simulink model "Fuel_Pump_V3_1_20201113_20KHz"  (R2019b)
settings: configuration reference "Configuration" (kept outside this file)
PreLoadFcn:
  | RTWConfigurationCB('preloadfcn', bdroot);
values from neighbouring files (symbols this model uses):
  MotorPara_Base_Frq = 666.0    [fuel_pump_V3_1_20201113_20kHz.sldd]
  MotorPara_Base_I = 50.0    [fuel_pump_V3_1_20201113_20kHz.sldd]
  MotorPara_Base_RPM = 12000.0    [fuel_pump_V3_1_20201113_20kHz.sldd]
  MotorPara_Base_V = 28.0    [fuel_pump_V3_1_20201113_20kHz.sldd]
  MotorPara_Ld = 1.287E-5    [fuel_pump_V3_1_20201113_20kHz.sldd]
  MotorPara_Lq = 2.052E-5    [fuel_pump_V3_1_20201113_20kHz.sldd]
  MotorPara_Ls = 8.3475E-5    [fuel_pump_V3_1_20201113_20kHz.sldd]
  MotorPara_P = 4.0    [fuel_pump_V3_1_20201113_20kHz.sldd]
  MotorPara_Rs = 0.01638    [fuel_pump_V3_1_20201113_20kHz.sldd]
  TPBRD_HALF = 1875.0    [fuel_pump_V3_1_20201113_20kHz.sldd]
  Ts_1kHz = 0.001    [fuel_pump_V3_1_20201113_20kHz.sldd]
  Ts_200Hz = 0.005    [fuel_pump_V3_1_20201113_20kHz.sldd]
  Ts_20KHz = 5.0E-5    [fuel_pump_V3_1_20201113_20kHz.sldd]
  Ts_40Hz = 0.025    [fuel_pump_V3_1_20201113_20kHz.sldd]
  Ts_50Hz = 0.02    [fuel_pump_V3_1_20201113_20kHz.sldd]
undefined symbols (not defined in the file or in its folder): DiscIntNeverNeededParam, Down, Up
libraries: c280xlib x22, c2833xlib x6, c2837xDlib x4, c28xdmclib x4, etargetslib x4, dspstat3 x2, c2000lib x1, idelinklib_common x1
(part 3 of 4)

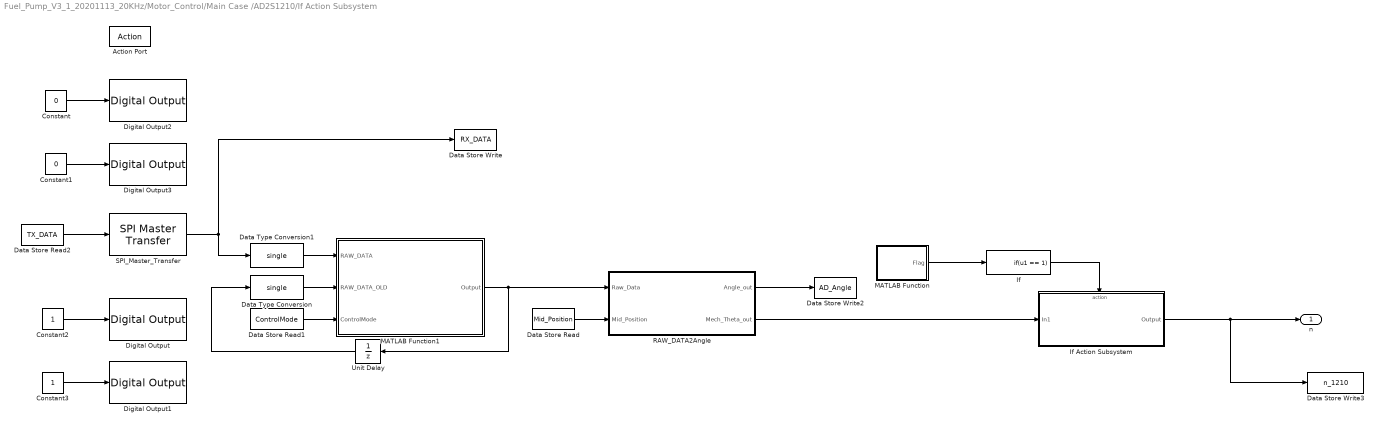
== system Fuel_Pump_V3_1_20201113_20KHz/Motor_Control/Main Case /AD2S1210/If Action Subsystem ==
  Action Port : ActionPort  ActionPortLabel=if(u1 > 0)
  Constant : Constant  Priority=1  Value=0  SampleTime=-1
  Constant1 : Constant  Priority=3  Value=0  SampleTime=-1
  Constant2 : Constant  Priority=11  SampleTime=-1
  Constant3 : Constant  Priority=12  SampleTime=-1
  Data Store Read : DataStoreRead  DataStoreName=Mid_Position
  Data Store Read1 : DataStoreRead  DataStoreName=ControlMode
  Data Store Read2 : DataStoreRead  Priority=5  DataStoreName=TX_DATA
  Data Store Write : DataStoreWrite  DataStoreName=RX_DATA
  Data Store Write2 : DataStoreWrite  DataStoreName=AD_Angle
  Data Store Write3 : DataStoreWrite  DataStoreName=n_1210
  Data Type Conversion : DataTypeConversion  OutDataTypeStr=single
  Data Type Conversion1 : DataTypeConversion  OutDataTypeStr=single
  Digital Output : c2837xDlib/Digital Output  GPIO_Number=GPIO16~GPIO23  GPIO_Bit0=off  GPIO_BIT0_Toggle=off  GPIO_Bit1=off  GPIO_BIT1_Toggle=off  GPIO_Bit2=off  GPIO_BIT2_Toggle=off  GPIO_Bit3=on  GPIO_BIT3_Toggle=off  GPIO_Bit4=off  GPIO_BIT4_Toggle=off  GPIO_Bit5=off  GPIO_BIT5_Toggle=off  GPIO_Bit6=off  GPIO_BIT6_Toggle=off  GPIO_Bit7=off  GPIO_BIT7_Toggle=off
      settings: SourceProductName=Embedded Coder Support Package for Texas Instruments C2000 Processors  SourceProductBaseCode=TIC2000
  Digital Output1 : c2837xDlib/Digital Output  GPIO_Number=GPIO16~GPIO23  GPIO_Bit0=off  GPIO_BIT0_Toggle=off  GPIO_Bit1=off  GPIO_BIT1_Toggle=off  GPIO_Bit2=off  GPIO_BIT2_Toggle=off  GPIO_Bit3=off  GPIO_BIT3_Toggle=off  GPIO_Bit4=on  GPIO_BIT4_Toggle=off  GPIO_Bit5=off  GPIO_BIT5_Toggle=off  GPIO_Bit6=off  GPIO_BIT6_Toggle=off  GPIO_Bit7=off  GPIO_BIT7_Toggle=off
      settings: SourceProductName=Embedded Coder Support Package for Texas Instruments C2000 Processors  SourceProductBaseCode=TIC2000
  Digital Output2 : c2837xDlib/Digital Output  GPIO_Number=GPIO16~GPIO23  GPIO_Bit0=off  GPIO_BIT0_Toggle=off  GPIO_Bit1=off  GPIO_BIT1_Toggle=off  GPIO_Bit2=off  GPIO_BIT2_Toggle=off  GPIO_Bit3=on  GPIO_BIT3_Toggle=off  GPIO_Bit4=off  GPIO_BIT4_Toggle=off  GPIO_Bit5=off  GPIO_BIT5_Toggle=off  GPIO_Bit6=off  GPIO_BIT6_Toggle=off  GPIO_Bit7=off  GPIO_BIT7_Toggle=off
      settings: SourceProductName=Embedded Coder Support Package for Texas Instruments C2000 Processors  SourceProductBaseCode=TIC2000
  Digital Output3 : c2837xDlib/Digital Output  GPIO_Number=GPIO16~GPIO23  GPIO_Bit0=off  GPIO_BIT0_Toggle=off  GPIO_Bit1=off  GPIO_BIT1_Toggle=off  GPIO_Bit2=off  GPIO_BIT2_Toggle=off  GPIO_Bit3=off  GPIO_BIT3_Toggle=off  GPIO_Bit4=on  GPIO_BIT4_Toggle=off  GPIO_Bit5=off  GPIO_BIT5_Toggle=off  GPIO_Bit6=off  GPIO_BIT6_Toggle=off  GPIO_Bit7=off  GPIO_BIT7_Toggle=off
      settings: SourceProductName=Embedded Coder Support Package for Texas Instruments C2000 Processors  SourceProductBaseCode=TIC2000
  If : If  IfExpression=u1 == 1  ShowElse=off
  If Action Subsystem : Subsystem  TreatAsAtomicUnit=on
  MATLAB Function : MATLAB Function  TreatAsAtomicUnit=on
  MATLAB Function1 : MATLAB Function  TreatAsAtomicUnit=on
  "RAW_DATA2Angle " : MATLAB Function  TreatAsAtomicUnit=on
  SPI_Master_Transfer : c280xlib/SPI Master Transfer  Priority=6  SPISelect=SPI_A  ClockPolarity=Rising_edge  ClockPhase=No_delay  SPIModule=uint32(0)  Mode=Master  BusSpeed=uint32(1000000)  FirstBitToTransfer=Most significant bit (MSB)  ClockMode=0  BlockFunction=Transfer  EnableRegisterAddress=off  RegisterAddress=255  OutputDataType=int8  OutputDataLength=1  DataBits=16  UseCustomSSPin=Provided by the SPI peripheral  ActiveLowSSPin=Active low  Pin=1
      settings: SourceProductName=Embedded Coder Support Package for Texas Instruments C2000 Processors  SourceProductBaseCode=TIC2000
  Unit Delay : UnitDelay  SampleTime=-1  HasFrameUpgradeWarning=on
  n : Outport
  wires:
  Constant1/1 -> Digital Output3/1
  Constant3/1 -> Digital Output1/1
  Constant/1 -> Digital Output2/1
  SPI_Master_Transfer/1 -> Data Type Conversion1/1, Data Store Write/1
  Constant2/1 -> Digital Output/1
  "RAW_DATA2Angle "/1(Angle_out) -> Data Store Write2/1
  Data Store Read2/1 -> SPI_Master_Transfer/1
  "RAW_DATA2Angle "/2(Mech_Theta_out) -> If Action Subsystem/1(In1)
  Data Store Read/1 -> "RAW_DATA2Angle "/2(Mid_Position)
  MATLAB Function/1(Flag) -> If/1
  If/1 -> If Action Subsystem/Action
  If Action Subsystem/1(Output) -> Data Store Write3/1, n/1
  MATLAB Function1/1(Output) -> "RAW_DATA2Angle "/1(Raw_Data), Unit Delay/1
  Unit Delay/1 -> Data Type Conversion/1
  Data Type Conversion/1 -> MATLAB Function1/2(RAW_DATA_OLD)
  Data Type Conversion1/1 -> MATLAB Function1/1(RAW_DATA)
  Data Store Read1/1 -> MATLAB Function1/3(ControlMode)

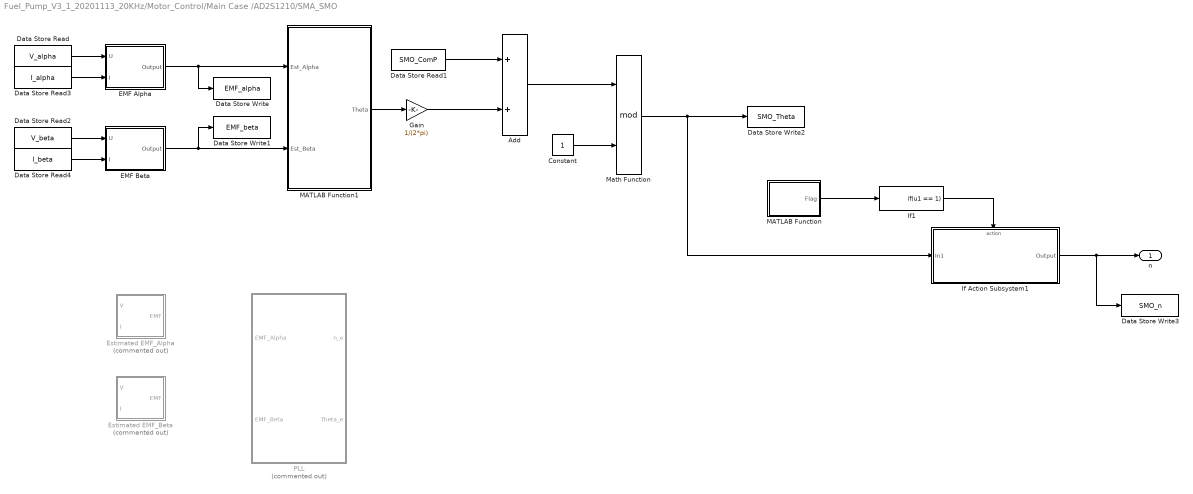
== system Fuel_Pump_V3_1_20201113_20KHz/Motor_Control/Main Case /AD2S1210/SMA_SMO ==
  Add : Sum
  Constant : Constant  OutDataTypeStr=single  SampleTime=-1
  Data Store Read : DataStoreRead  DataStoreName=V_alpha
  Data Store Read1 : DataStoreRead  DataStoreName=SMO_ComP
  Data Store Read2 : DataStoreRead  DataStoreName=V_beta
  Data Store Read3 : DataStoreRead  DataStoreName=I_alpha
  Data Store Read4 : DataStoreRead  DataStoreName=I_beta
  Data Store Write : DataStoreWrite  DataStoreName=EMF_alpha
  Data Store Write1 : DataStoreWrite  DataStoreName=EMF_beta
  Data Store Write2 : DataStoreWrite  DataStoreName=SMO_Theta
  Data Store Write3 : DataStoreWrite  DataStoreName=SMO_n
  EMF Alpha : Subsystem
  EMF Beta : Subsystem
  Estimated EMF_Alpha : Subsystem  Commented=on
  Estimated EMF_Beta : Subsystem  Commented=on
  Gain : Gain  Gain=1/(2*pi)
  If Action Subsystem1 : Subsystem  TreatAsAtomicUnit=on
  If1 : If  IfExpression=u1 == 1  ShowElse=off
  MATLAB Function : MATLAB Function  TreatAsAtomicUnit=on
  MATLAB Function1 : MATLAB Function  TreatAsAtomicUnit=on
  Math Function : Math  Operator=mod  SignedPower=off  SaturateOnIntegerOverflow=on
  PLL : Subsystem  Commented=on
  n : Outport
  wires:
  If Action Subsystem1/1(Output) -> Data Store Write3/1, n/1
  MATLAB Function/1(Flag) -> If1/1
  Data Store Read3/1 -> EMF Alpha/2(I)
  EMF Alpha/1(Output) -> MATLAB Function1/1(Est_Alpha), Data Store Write/1
  Data Store Read/1 -> EMF Alpha/1(U)
  EMF Beta/1(Output) -> MATLAB Function1/2(Est_Beta), Data Store Write1/1
  If1/1 -> If Action Subsystem1/Action
  Data Store Read4/1 -> EMF Beta/2(I)
  Data Store Read2/1 -> EMF Beta/1(U)
  Constant/1 -> Math Function/2
  Data Store Read1/1 -> Add/1
  Add/1 -> Math Function/1
  MATLAB Function1/1(Theta) -> Gain/1
  Gain/1 -> Add/2
  Math Function/1 -> If Action Subsystem1/1(In1), Data Store Write2/1

== system Fuel_Pump_V3_1_20201113_20KHz/Motor_Control/Main Case /Current_PI/PID_Id  ==
  Ref : Inport
  Fbk : Inport  Port=2
  Data Store Read : DataStoreRead  DataStoreName=PK_KpId
  Data Store Read1 : DataStoreRead  DataStoreName=uiId
  Data Store Write : DataStoreWrite  DataStoreName=uiId
  "Integral " : Subsystem
  Product : Product  OutDataTypeStr=Inherit: Same as first input
  Saturation : Saturate  UpperLimit=MotorPara_Base_V  LowerLimit=-MotorPara_Base_V
  Sum1 : Sum
  Sum2 : Sum  Inputs=+-  OutDataTypeStr=Inherit: Inherit via back propagation
  Out : Outport
  wires:
  Data Store Read1/1 -> "Integral "/1(OLD_UI)
  Fbk/1 -> Sum2/2
  Ref/1 -> Sum2/1
  Product/1 -> Sum1/1
  Data Store Read/1 -> Product/2
  "Integral "/1(UI) -> Data Store Write/1, Sum1/2
  Sum2/1 -> "Integral "/2(UP), Product/1
  Sum1/1 -> Saturation/1
  Saturation/1 -> Out/1

== system Fuel_Pump_V3_1_20201113_20KHz/Motor_Control/Main Case /Current_PI/PID_Iq ==
  Ref : Inport
  Fbk : Inport  Port=2
  Data Store Read : DataStoreRead  DataStoreName=PK_KpIq
  Data Store Read1 : DataStoreRead  DataStoreName=uiIq
  Data Store Write : DataStoreWrite  DataStoreName=uiIq
  "Integral " : Subsystem
  Product : Product  OutDataTypeStr=Inherit: Same as first input
  Saturation : Saturate  UpperLimit=MotorPara_Base_V  LowerLimit=-MotorPara_Base_V
  Sum1 : Sum
  Sum2 : Sum  Inputs=+-  OutDataTypeStr=Inherit: Inherit via back propagation
  Out : Outport
  wires:
  Data Store Read1/1 -> "Integral "/1(OLD_UI)
  Fbk/1 -> Sum2/2
  Ref/1 -> Sum2/1
  Product/1 -> Sum1/1
  Data Store Read/1 -> Product/2
  "Integral "/1(UI) -> Data Store Write/1, Sum1/2
  Sum2/1 -> "Integral "/2(UP), Product/1
  Sum1/1 -> Saturation/1
  Saturation/1 -> Out/1

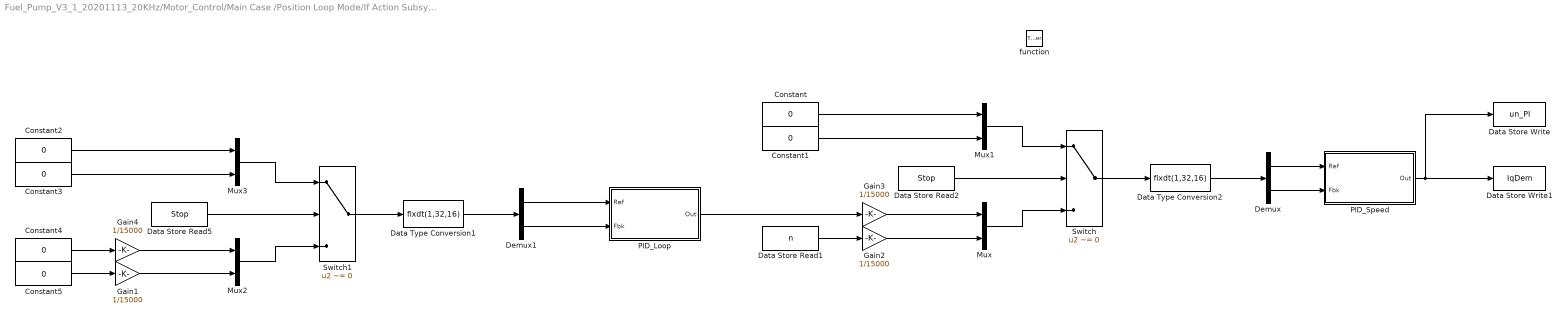
== system Fuel_Pump_V3_1_20201113_20KHz/Motor_Control/Main Case /Position Loop Mode/If Action Subsystem ==
  function : TriggerPort  TriggerType=function-call  VariantControl=Variant
  Constant{,1..5} (6 alike) : Constant  Value=0  OutDataTypeStr=single  SampleTime=-1
  Data Store Read1 : DataStoreRead  DataStoreName=n
  Data Store Read2 : DataStoreRead  DataStoreName=Stop
  Data Store Read5 : DataStoreRead  DataStoreName=Stop
  Data Store Write : DataStoreWrite  DataStoreName=un_PI
  Data Store Write1 : DataStoreWrite  DataStoreName=IqDem
  Data Type Conversion1 : DataTypeConversion  OutDataTypeStr=fixdt(1,32,16)
  Data Type Conversion2 : DataTypeConversion  OutDataTypeStr=fixdt(1,32,16)
  Demux : Demux  Outputs=2
  Demux1 : Demux  Outputs=2
  Gain{1..4} (4 alike) : Gain  Gain=1/15000  OutDataTypeStr=Inherit: Inherit via back propagation
  Mux{,1..3} (4 alike) : Mux  Inputs=2
  PID_Loop : Subsystem
  PID_Speed : Subsystem
  Switch : Switch  Criteria=u2 ~= 0
  Switch1 : Switch  Criteria=u2 ~= 0
  wires:
  PID_Speed/1(Out) -> Data Store Write1/1, Data Store Write/1
  Demux/1 -> PID_Speed/1(Ref)
  Demux/2 -> PID_Speed/2(Fbk)
  Switch/1 -> Data Type Conversion2/1
  Data Store Read2/1 -> Switch/2
  Gain3/1 -> Mux/1
  Data Store Read1/1 -> Gain2/1
  PID_Loop/1(Out) -> Gain3/1
  Gain2/1 -> Mux/2
  Mux1/1 -> Switch/1
  Mux/1 -> Switch/3
  Constant/1 -> Mux1/1
  Constant1/1 -> Mux1/2
  Data Type Conversion2/1 -> Demux/1
  Data Store Read5/1 -> Switch1/2
  Constant3/1 -> Mux3/2
  Data Type Conversion1/1 -> Demux1/1
  Mux3/1 -> Switch1/1
  Gain1/1 -> Mux2/2
  Constant2/1 -> Mux3/1
  Constant5/1 -> Gain1/1
  Gain4/1 -> Mux2/1
  Constant4/1 -> Gain4/1
  Switch1/1 -> Data Type Conversion1/1
  Demux1/1 -> PID_Loop/1(Ref)
  Mux2/1 -> Switch1/3
  Demux1/2 -> PID_Loop/2(Fbk)

== system Fuel_Pump_V3_1_20201113_20KHz/Motor_Control/Main Case /SVPWM/Inverse Park Transformation ==
  D : Inport
  Q : Inport  Port=2
  theta : Inport  Port=3
  Gain : Gain  Gain=2*pi
  Product{,1..3} (4 alike) : Product  OutDataTypeStr=Inherit: Same as first input
  Sin : Trigonometry  OutputSignalType=real
  Sin1 : Trigonometry  Operator=cos  OutputSignalType=real
  Sum1 : Sum  Inputs=|++  OutDataTypeStr=Inherit: Same as first input
  Sum2 : Sum  Inputs=|+-  OutDataTypeStr=Inherit: Same as first input
  Alpha : Outport
  Beta : Outport  Port=2
  wires:
  Sin1/1 -> Product2/2, Product/2
  Sin/1 -> Product3/2, Product1/2
  Product3/1 -> Sum1/2
  Sum1/1 -> Beta/1
  D/1 -> Product3/1, Product/1
  Product2/1 -> Sum1/1
  Sum2/1 -> Alpha/1
  Product/1 -> Sum2/1
  Product1/1 -> Sum2/2
  theta/1 -> Gain/1
  Q/1 -> Product2/1, Product1/1
  Gain/1 -> Sin/1, Sin1/1

== system Fuel_Pump_V3_1_20201113_20KHz/Motor_Control/Main Case /Speed Loop Mode/If Action Subsystem ==
  function : TriggerPort  TriggerType=function-call  VariantControl=Variant
  Constant : Constant  Value=0  OutDataTypeStr=single  SampleTime=-1
  Constant1 : Constant  Value=0  OutDataTypeStr=single  SampleTime=-1
  Data Store Read1 : DataStoreRead  DataStoreName=n
  Data Store Read2 : DataStoreRead  DataStoreName=Stop
  Data Store Read3 : DataStoreRead  DataStoreName=nDem_PI
  Data Store Write1 : DataStoreWrite  DataStoreName=IqDem
  Demux : Demux  Outputs=2
  Mux : Mux  Inputs=2
  Mux1 : Mux  Inputs=2
  "PID_n " : Subsystem
  Switch : Switch  Criteria=u2 ~= 0
  wires:
  "PID_n "/1(Out) -> Data Store Write1/1
  Demux/1 -> "PID_n "/1(Ref)
  Demux/2 -> "PID_n "/2(Fbk)
  Data Store Read2/1 -> Switch/2
  Data Store Read3/1 -> Mux/1
  Data Store Read1/1 -> Mux/2
  Mux1/1 -> Switch/1
  Mux/1 -> Switch/3
  Constant/1 -> Mux1/1
  Constant1/1 -> Mux1/2
  Switch/1 -> Demux/1

== system Fuel_Pump_V3_1_20201113_20KHz/Motor_Control/Main Case /AD2S1210/If Action Subsystem/If Action Subsystem ==
  In1 : Inport
  Action Port : ActionPort  ActionPortLabel=if(u1 == 1)
  Delay1 : Delay  DelayLength=1
  First Order Filter : Subsystem
  MATLAB Function1 : MATLAB Function  TreatAsAtomicUnit=on
  Output : Outport
  wires:
  In1/1 -> Delay1/1, MATLAB Function1/1(theta)
  Delay1/1 -> MATLAB Function1/2(theta_old)
  First Order Filter/1("output ") -> Output/1
  MATLAB Function1/1(speed) -> First Order Filter/1(input)

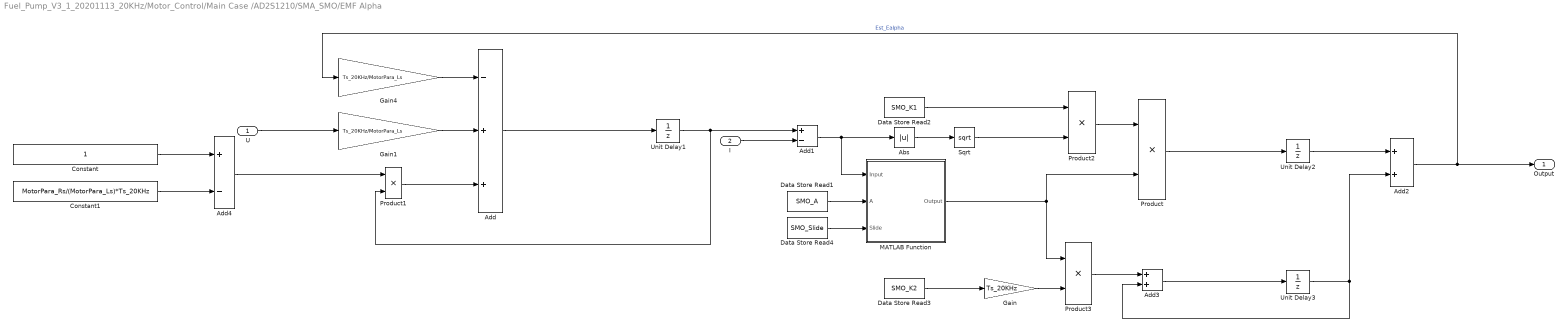
== system Fuel_Pump_V3_1_20201113_20KHz/Motor_Control/Main Case /AD2S1210/SMA_SMO/EMF Alpha ==
  U : Inport
  I : Inport  Port=2
  Abs : Abs
  Add : Sum  Inputs=-++
  Add1 : Sum  Inputs=+-  OutDataTypeStr=Inherit: Inherit via back propagation
  Add2 : Sum
  Add3 : Sum
  Add4 : Sum  Inputs=+-
  Constant : Constant  OutDataTypeStr=single  SampleTime=-1
  Constant1 : Constant  Value=MotorPara_Rs/(MotorPara_Ls)*Ts_20KHz  OutDataTypeStr=single  SampleTime=-1
  Data Store Read1 : DataStoreRead  DataStoreName=SMO_A
  Data Store Read2 : DataStoreRead  DataStoreName=SMO_K1
  Data Store Read3 : DataStoreRead  DataStoreName=SMO_K2
  Data Store Read4 : DataStoreRead  DataStoreName=SMO_Slide
  Gain : Gain  Gain=Ts_20KHz
  Gain1 : Gain  Gain=Ts_20KHz/MotorPara_Ls  OutDataTypeStr=Inherit: Inherit via back propagation
  Gain4 : Gain  Gain=Ts_20KHz/MotorPara_Ls  OutDataTypeStr=Inherit: Inherit via back propagation
  MATLAB Function : MATLAB Function  TreatAsAtomicUnit=on
  Product{,1..3} (4 alike) : Product
  Sqrt : Sqrt  SaturateOnIntegerOverflow=on
  Unit Delay1 : UnitDelay  SampleTime=-1  HasFrameUpgradeWarning=on
  Unit Delay2 : UnitDelay  SampleTime=-1  HasFrameUpgradeWarning=on
  Unit Delay3 : UnitDelay  SampleTime=-1  HasFrameUpgradeWarning=on
  Output : Outport
  wires:
  Product3/1 -> Add3/1
  Gain4/1 -> Add/1
  Gain1/1 -> Add/2
  Add2/1 -> Output/1, Gain4/1  "Est_Ealpha"
  Product1/1 -> Add/3
  Product2/1 -> Product/1
  Sqrt/1 -> Product2/2
  U/1 -> Gain1/1
  I/1 -> Add1/2
  Add1/1 -> MATLAB Function/1(Input), Abs/1
  Abs/1 -> Sqrt/1
  Unit Delay2/1 -> Add2/1
  Add4/1 -> Product1/1
  Constant/1 -> Add4/1
  Constant1/1 -> Add4/2
  Data Store Read1/1 -> MATLAB Function/2(A)
  Data Store Read2/1 -> Product2/1
  Gain/1 -> Product3/2
  Data Store Read3/1 -> Gain/1
  Unit Delay1/1 -> Product1/2, Add1/1
  Unit Delay3/1 -> Add3/2, Add2/2
  Add/1 -> Unit Delay1/1
  MATLAB Function/1(Output) -> Product/2, Product3/1
  Product/1 -> Unit Delay2/1
  Add3/1 -> Unit Delay3/1
  Data Store Read4/1 -> MATLAB Function/3(Slide)

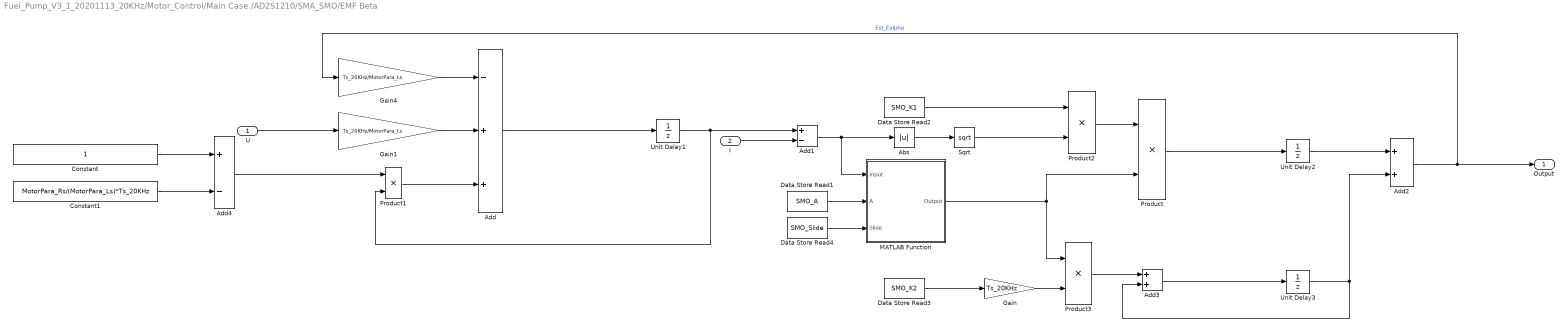
== system Fuel_Pump_V3_1_20201113_20KHz/Motor_Control/Main Case /AD2S1210/SMA_SMO/EMF Beta ==
  U : Inport
  I : Inport  Port=2
  Abs : Abs
  Add : Sum  Inputs=-++
  Add1 : Sum  Inputs=+-  OutDataTypeStr=Inherit: Inherit via back propagation
  Add2 : Sum
  Add3 : Sum
  Add4 : Sum  Inputs=+-
  Constant : Constant  OutDataTypeStr=single  SampleTime=-1
  Constant1 : Constant  Value=MotorPara_Rs/(MotorPara_Ls)*Ts_20KHz  OutDataTypeStr=single  SampleTime=-1
  Data Store Read1 : DataStoreRead  DataStoreName=SMO_A
  Data Store Read2 : DataStoreRead  DataStoreName=SMO_K1
  Data Store Read3 : DataStoreRead  DataStoreName=SMO_K2
  Data Store Read4 : DataStoreRead  DataStoreName=SMO_Slide
  Gain : Gain  Gain=Ts_20KHz
  Gain1 : Gain  Gain=Ts_20KHz/MotorPara_Ls  OutDataTypeStr=Inherit: Inherit via back propagation
  Gain4 : Gain  Gain=Ts_20KHz/MotorPara_Ls  OutDataTypeStr=Inherit: Inherit via back propagation
  MATLAB Function : MATLAB Function  TreatAsAtomicUnit=on
  Product{,1..3} (4 alike) : Product
  Sqrt : Sqrt  SaturateOnIntegerOverflow=on
  Unit Delay1 : UnitDelay  SampleTime=-1  HasFrameUpgradeWarning=on
  Unit Delay2 : UnitDelay  SampleTime=-1  HasFrameUpgradeWarning=on
  Unit Delay3 : UnitDelay  SampleTime=-1  HasFrameUpgradeWarning=on
  Output : Outport
  wires:
  Data Store Read4/1 -> MATLAB Function/3(Slide)
  Add3/1 -> Unit Delay3/1
  Product/1 -> Unit Delay2/1
  MATLAB Function/1(Output) -> Product3/1, Product/2
  Add/1 -> Unit Delay1/1
  Unit Delay3/1 -> Add2/2, Add3/2
  Unit Delay1/1 -> Add1/1, Product1/2
  Data Store Read3/1 -> Gain/1
  Gain/1 -> Product3/2
  Data Store Read2/1 -> Product2/1
  Data Store Read1/1 -> MATLAB Function/2(A)
  Constant1/1 -> Add4/2
  Constant/1 -> Add4/1
  Add4/1 -> Product1/1
  Unit Delay2/1 -> Add2/1
  Abs/1 -> Sqrt/1
  Add1/1 -> Abs/1, MATLAB Function/1(Input)
  I/1 -> Add1/2
  U/1 -> Gain1/1
  Sqrt/1 -> Product2/2
  Product2/1 -> Product/1
  Product1/1 -> Add/3
  Add2/1 -> Gain4/1, Output/1  "Est_Ealpha"
  Gain1/1 -> Add/2
  Gain4/1 -> Add/1
  Product3/1 -> Add3/1

== system Fuel_Pump_V3_1_20201113_20KHz/Motor_Control/Main Case /AD2S1210/SMA_SMO/Estimated EMF_Alpha ==
  V : Inport
  I : Inport  Port=2
  Add : Sum  Inputs=+--
  Add1 : Sum
  Add2 : Sum  Inputs=+-
  Data Store Read1 : DataStoreRead  DataStoreName=SMO_Slide
  Data Store Read2 : DataStoreRead  DataStoreName=SMO_A
  First Order Filter : Subsystem
  Gain2 : Gain  Gain=exp(-MotorPara_Rs*Ts_20KHz/MotorPara_Ls)
  Gain3 : Gain  Gain=(1/MotorPara_Rs)*(1-exp(-MotorPara_Rs*Ts_20KHz/MotorPara_Ls))
  MATLAB Function : MATLAB Function  TreatAsAtomicUnit=on
  Unit Delay : UnitDelay  SampleTime=-1  HasFrameUpgradeWarning=on
  Unit Delay1 : UnitDelay  SampleTime=-1  HasFrameUpgradeWarning=on
  Unit Delay2 : UnitDelay  SampleTime=-1  HasFrameUpgradeWarning=on
  EMF : Outport
  wires:
  First Order Filter/1("output ") -> EMF/1, Unit Delay2/1
  Gain2/1 -> Add1/2
  Add1/1 -> Unit Delay/1, Add2/1  "Est_Ialpha"
  Gain3/1 -> Add1/1
  MATLAB Function/1(output) -> Unit Delay1/1, First Order Filter/1(input)
  Data Store Read1/1 -> MATLAB Function/2(slide)
  Add/1 -> Gain3/1
  Add2/1 -> MATLAB Function/1(input)
  Unit Delay/1 -> Gain2/1  "Est_Ialpha_old"
  I/1 -> Add2/2
  Unit Delay1/1 -> Add/3  "Zalpha_old"
  Unit Delay2/1 -> Add/2  "Ealpha_old"
  V/1 -> Add/1
  Data Store Read2/1 -> MATLAB Function/3(E0)

== system Fuel_Pump_V3_1_20201113_20KHz/Motor_Control/Main Case /AD2S1210/SMA_SMO/Estimated EMF_Beta ==
  V : Inport
  I : Inport  Port=2
  Add : Sum  Inputs=+--
  Add1 : Sum
  Add2 : Sum  Inputs=+-
  Data Store Read1 : DataStoreRead  DataStoreName=SMO_Slide
  Data Store Read2 : DataStoreRead  DataStoreName=SMO_A
  First Order Filter : Subsystem
  Gain2 : Gain  Gain=exp(-MotorPara_Rs*Ts_20KHz/MotorPara_Ls)
  Gain3 : Gain  Gain=(1/MotorPara_Rs)*(1-exp(-MotorPara_Rs*Ts_20KHz/MotorPara_Ls))
  MATLAB Function : MATLAB Function  TreatAsAtomicUnit=on
  Unit Delay : UnitDelay  SampleTime=-1  HasFrameUpgradeWarning=on
  Unit Delay1 : UnitDelay  SampleTime=-1  HasFrameUpgradeWarning=on
  Unit Delay2 : UnitDelay  SampleTime=-1  HasFrameUpgradeWarning=on
  EMF : Outport
  wires:
  Data Store Read2/1 -> MATLAB Function/3(E0)
  V/1 -> Add/1
  Unit Delay2/1 -> Add/2  "Ealpha_old"
  Unit Delay1/1 -> Add/3  "Zalpha_old"
  I/1 -> Add2/2
  Unit Delay/1 -> Gain2/1  "Est_Ialpha_old"
  Add2/1 -> MATLAB Function/1(input)
  Add/1 -> Gain3/1
  Data Store Read1/1 -> MATLAB Function/2(slide)
  MATLAB Function/1(output) -> First Order Filter/1(input), Unit Delay1/1
  Gain3/1 -> Add1/1
  Add1/1 -> Add2/1, Unit Delay/1  "Est_Ialpha"
  Gain2/1 -> Add1/2
  First Order Filter/1("output ") -> Unit Delay2/1, EMF/1

== system Fuel_Pump_V3_1_20201113_20KHz/Motor_Control/Main Case /AD2S1210/SMA_SMO/If Action Subsystem1 ==
  In1 : Inport
  Action Port : ActionPort  ActionPortLabel=if(u1 == 1)
  Data Store Read : DataStoreRead  DataStoreName=n_R
  Data Store Read1 : DataStoreRead  DataStoreName=n_Q
  Delay1 : Delay  DelayLength=1
  First Order Filter : Subsystem  Commented=on
  Kalman_Filter : MATLAB Function  TreatAsAtomicUnit=on
  MATLAB Function1 : MATLAB Function  TreatAsAtomicUnit=on
  Output : Outport
  wires:
  In1/1 -> Delay1/1, MATLAB Function1/1(theta)
  MATLAB Function1/1(speed) -> Kalman_Filter/1(Input)
  Delay1/1 -> MATLAB Function1/2(theta_old)
  Kalman_Filter/1(optimal_value_out) -> Output/1
  Data Store Read1/1 -> Kalman_Filter/2(n_Q)
  Data Store Read/1 -> Kalman_Filter/3(n_R)

== system Fuel_Pump_V3_1_20201113_20KHz/Motor_Control/Main Case /AD2S1210/SMA_SMO/PLL ==
  EMF_Alpha : Inport
  EMF_Beta : Inport  Port=2
  Add : Sum  Inputs=+-
  Add1 : Sum
  Constant : Constant  Value=2*pi  OutDataTypeStr=single  SampleTime=-1
  Constant1 : Constant  OutDataTypeStr=single  SampleTime=-1
  Data Store Read : DataStoreRead  DataStoreName=SMO_ComP
  Discrete-Time Integrator : DiscreteIntegrator  SampleTime=-1  OutDataTypeStr=single  ICPrevOutput=DiscIntNeverNeededParam  ICPrevScaledInput=DiscIntNeverNeededParam
  Gain : Gain  Gain=-1
  Gain1 : Gain  Gain=1/(2*pi)
  Math Function : Math  Operator=mod  SignedPower=off  OutputSignalType=real  SaturateOnIntegerOverflow=on
  Math Function1 : Math  Operator=mod  SignedPower=off  OutputSignalType=real  SaturateOnIntegerOverflow=on
  "PLL_PI " : Subsystem
  Product : Product
  Product1 : Product
  Sin : Trigonometry  OutputSignalType=real
  Sin1 : Trigonometry  Operator=cos  OutputSignalType=real
  n_e : Outport
  Theta_e : Outport  Port=2
  wires:
  EMF_Alpha/1 -> Gain/1
  Gain/1 -> Product/2
  EMF_Beta/1 -> Product1/1
  Product/1 -> Add/1
  Product1/1 -> Add/2
  Discrete-Time Integrator/1 -> Math Function/1
  Math Function/1 -> Sin/1, Gain1/1, Sin1/1
  Constant/1 -> Math Function/2
  Sin1/1 -> Product/1
  Sin/1 -> Product1/2
  Add/1 -> "PLL_PI "/1(Ref)
  "PLL_PI "/1(Out) -> n_e/1, Discrete-Time Integrator/1
  Gain1/1 -> Add1/1
  Data Store Read/1 -> Add1/2
  Constant1/1 -> Math Function1/2
  Add1/1 -> Math Function1/1
  Math Function1/1 -> Theta_e/1

== system Fuel_Pump_V3_1_20201113_20KHz/Motor_Control/Main Case /Current_PI/PID_Id /Integral  ==
  OLD_UI : Inport
  UP : Inport  Port=2
  Data Store Read2 : DataStoreRead  DataStoreName=PK_KiId
  Gain : Gain  Gain=Ts_20KHz
  Product1 : Product  OutDataTypeStr=Inherit: Same as first input
  Sum3 : Sum
  UI : Outport
  wires:
  Sum3/1 -> UI/1
  UP/1 -> Product1/2
  Product1/1 -> Sum3/2
  OLD_UI/1 -> Sum3/1
  Data Store Read2/1 -> Gain/1
  Gain/1 -> Product1/1

== system Fuel_Pump_V3_1_20201113_20KHz/Motor_Control/Main Case /Current_PI/PID_Iq/Integral  ==
  OLD_UI : Inport
  UP : Inport  Port=2
  Data Store Read2 : DataStoreRead  DataStoreName=PK_KiIq
  Gain : Gain  Gain=Ts_20KHz
  Product1 : Product  OutDataTypeStr=Inherit: Same as first input
  Sum3 : Sum
  UI : Outport
  wires:
  Sum3/1 -> UI/1
  UP/1 -> Product1/2
  Product1/1 -> Sum3/2
  OLD_UI/1 -> Sum3/1
  Data Store Read2/1 -> Gain/1
  Gain/1 -> Product1/1

== system Fuel_Pump_V3_1_20201113_20KHz/Motor_Control/Main Case /Position Loop Mode/If Action Subsystem/PID_Loop ==
  Ref : Inport
  Fbk : Inport  Port=2
  " " : etargetslib/ 
      settings: SourceProductName=MATLAB Coder  SourceProductBaseCode=ME
  " 1" : etargetslib/ 
      settings: SourceProductName=MATLAB Coder  SourceProductBaseCode=ME
  Data Store Read : DataStoreRead  DataStoreName=PK_Kpn
  Data Store Read1 : DataStoreRead  DataStoreName=uin
  Data Store Write : DataStoreWrite  DataStoreName=en
  Data Store Write1 : DataStoreWrite  DataStoreName=uin
  Data Type Conversion{,1..2,5} (4 alike) : DataTypeConversion
  Product : Product  OutDataTypeStr=Inherit: Same as first input
  Saturation : Saturate  UpperLimit=1  LowerLimit=-1  OutDataTypeStr=Inherit: Inherit via back propagation
  Saturation1 : Saturate  UpperLimit=1  LowerLimit=-1  OutDataTypeStr=fixdt(1,32,16)
  Sum1 : Sum
  Sum2 : Sum  Inputs=+-  OutDataTypeStr=fixdt(1,32,16)
  UI_REG3 : Subsystem  AncestorBlock=c28xdmclib/PID Controller/UI_REG3
  Out : Outport
  wires:
  Data Type Conversion2/1 -> UI_REG3/1(OLD_UI_REG3)
  Data Type Conversion1/1 -> Data Store Write1/1
  UI_REG3/1(UI_REG1) -> Saturation1/1
  Sum1/1 -> Saturation/1
  Data Type Conversion5/1 -> Data Store Write/1
  Saturation/1 -> Out/1
  Saturation1/1 -> Sum1/2, Data Type Conversion1/1
  Data Type Conversion/1 -> Product/2
  Fbk/1 -> " 1"/1
  Data Store Read1/1 -> Data Type Conversion2/1
  Ref/1 -> " "/1
  Sum2/1 -> Product/1, Data Type Conversion5/1
  " 1"/1 -> Sum2/2
  " "/1 -> Sum2/1
  Product/1 -> UI_REG3/2(up_reg3), Sum1/1
  Data Store Read/1 -> Data Type Conversion/1

== system Fuel_Pump_V3_1_20201113_20KHz/Motor_Control/Main Case /Position Loop Mode/If Action Subsystem/PID_Speed ==
  Ref : Inport
  Fbk : Inport  Port=2
  " " : etargetslib/ 
      settings: SourceProductName=MATLAB Coder  SourceProductBaseCode=ME
  " 1" : etargetslib/ 
      settings: SourceProductName=MATLAB Coder  SourceProductBaseCode=ME
  Data Store Read : DataStoreRead  DataStoreName=PK_Kpn
  Data Store Read1 : DataStoreRead  DataStoreName=uin
  Data Store Write : DataStoreWrite  DataStoreName=en
  Data Store Write1 : DataStoreWrite  DataStoreName=uin
  Data Type Conversion{,1..2,5} (4 alike) : DataTypeConversion
  Product : Product  OutDataTypeStr=Inherit: Same as first input
  Saturation : Saturate  UpperLimit=1  LowerLimit=-1  OutDataTypeStr=Inherit: Inherit via back propagation
  Saturation1 : Saturate  UpperLimit=1  LowerLimit=-1  OutDataTypeStr=fixdt(1,32,16)
  Sum1 : Sum
  Sum2 : Sum  Inputs=+-  OutDataTypeStr=fixdt(1,32,16)
  UI_REG3 : Subsystem  AncestorBlock=c28xdmclib/PID Controller/UI_REG3
  Out : Outport
  wires:
  Data Store Read/1 -> Data Type Conversion/1
  Product/1 -> Sum1/1, UI_REG3/2(up_reg3)
  " "/1 -> Sum2/1
  " 1"/1 -> Sum2/2
  Sum2/1 -> Data Type Conversion5/1, Product/1
  Ref/1 -> " "/1
  Data Store Read1/1 -> Data Type Conversion2/1
  Fbk/1 -> " 1"/1
  Data Type Conversion/1 -> Product/2
  Saturation1/1 -> Data Type Conversion1/1, Sum1/2
  Saturation/1 -> Out/1
  Data Type Conversion5/1 -> Data Store Write/1
  Sum1/1 -> Saturation/1
  UI_REG3/1(UI_REG1) -> Saturation1/1
  Data Type Conversion1/1 -> Data Store Write1/1
  Data Type Conversion2/1 -> UI_REG3/1(OLD_UI_REG3)

== system Fuel_Pump_V3_1_20201113_20KHz/Motor_Control/Main Case /Speed Loop Mode/If Action Subsystem/PID_n  ==
  Ref : Inport
  Fbk : Inport  Port=2
  Data Store Read : DataStoreRead  DataStoreName=PK_Kpn
  Data Store Read1 : DataStoreRead  DataStoreName=uin
  Data Store Write : DataStoreWrite  DataStoreName=uin
  "Integral " : Subsystem
  Product : Product  OutDataTypeStr=Inherit: Same as first input
  Saturation : Saturate  UpperLimit=MotorPara_Base_I*1.5  LowerLimit=-MotorPara_Base_I*1.5
  Sum1 : Sum
  Sum2 : Sum  Inputs=+-  OutDataTypeStr=Inherit: Inherit via back propagation
  Out : Outport
  wires:
  Data Store Read1/1 -> "Integral "/1(OLD_UI)
  Fbk/1 -> Sum2/2
  Ref/1 -> Sum2/1
  Product/1 -> Sum1/1
  Data Store Read/1 -> Product/2
  "Integral "/1(UI) -> Data Store Write/1, Sum1/2
  Sum2/1 -> "Integral "/2(UP), Product/1
  Sum1/1 -> Saturation/1
  Saturation/1 -> Out/1

== system Fuel_Pump_V3_1_20201113_20KHz/Motor_Control/Main Case /AD2S1210/If Action Subsystem/If Action Subsystem/First Order Filter ==
  input : Inport
  Add : Sum  Inputs=+-
  Add3 : Sum  AccumDataTypeStr=single
  Constant : Constant  OutDataTypeStr=single  SampleTime=-1
  Data Store Read1 : DataStoreRead  DataStoreName=n_Filter
  Data Store Read2 : DataStoreRead  DataStoreName=n_Filter
  Gain : Gain  Gain=2*pi*Ts_20KHz*20
  Gain1 : Gain  Gain=2*pi*Ts_20KHz*20
  Product : Product
  Product1 : Product
  Unit Delay3 : UnitDelay  SampleTime=-1  HasFrameUpgradeWarning=on
  "output " : Outport
  wires:
  input/1 -> Product/1
  Product/1 -> Add3/1
  Product1/1 -> Unit Delay3/1
  Add3/1 -> Product1/1, "output "/1
  Unit Delay3/1 -> Add3/2
  Data Store Read2/1 -> Gain/1
  Gain/1 -> Product/2
  Data Store Read1/1 -> Gain1/1
  Add/1 -> Product1/2
  Gain1/1 -> Add/2
  Constant/1 -> Add/1

== system Fuel_Pump_V3_1_20201113_20KHz/Motor_Control/Main Case /AD2S1210/SMA_SMO/Estimated EMF_Alpha/First Order Filter ==
  input : Inport
  Add : Sum  Inputs=+-
  Add3 : Sum  AccumDataTypeStr=single
  Constant : Constant  OutDataTypeStr=single
  Data Store Read1 : DataStoreRead  DataStoreName=SMO_Filter
  Data Store Read2 : DataStoreRead  DataStoreName=SMO_Filter
  Gain : Gain  Gain=MotorPara_P/60*2*pi*Ts_20KHz
  Gain1 : Gain  Gain=MotorPara_P/60*2*pi*Ts_20KHz
  Product : Product
  Product1 : Product
  Unit Delay3 : UnitDelay  SampleTime=-1  HasFrameUpgradeWarning=on
  "output " : Outport
  wires:
  input/1 -> Product/1
  Product/1 -> Add3/1
  Product1/1 -> Unit Delay3/1
  Add3/1 -> Product1/1, "output "/1
  Unit Delay3/1 -> Add3/2
  Data Store Read2/1 -> Gain/1
  Gain/1 -> Product/2
  Data Store Read1/1 -> Gain1/1
  Add/1 -> Product1/2
  Gain1/1 -> Add/2
  Constant/1 -> Add/1

== system Fuel_Pump_V3_1_20201113_20KHz/Motor_Control/Main Case /AD2S1210/SMA_SMO/Estimated EMF_Beta/First Order Filter ==
  input : Inport
  Add : Sum  Inputs=+-
  Add3 : Sum  AccumDataTypeStr=single
  Constant : Constant  OutDataTypeStr=single
  Data Store Read1 : DataStoreRead  DataStoreName=SMO_Filter
  Data Store Read2 : DataStoreRead  DataStoreName=SMO_Filter
  Gain : Gain  Gain=MotorPara_P/60*2*pi*Ts_20KHz
  Gain1 : Gain  Gain=MotorPara_P/60*2*pi*Ts_20KHz
  Product : Product
  Product1 : Product
  Unit Delay3 : UnitDelay  SampleTime=-1  HasFrameUpgradeWarning=on
  "output " : Outport
  wires:
  Constant/1 -> Add/1
  Gain1/1 -> Add/2
  Add/1 -> Product1/2
  Data Store Read1/1 -> Gain1/1
  Gain/1 -> Product/2
  Data Store Read2/1 -> Gain/1
  Unit Delay3/1 -> Add3/2
  Add3/1 -> "output "/1, Product1/1
  Product1/1 -> Unit Delay3/1
  Product/1 -> Add3/1
  input/1 -> Product/1

== system Fuel_Pump_V3_1_20201113_20KHz/Motor_Control/Main Case /AD2S1210/SMA_SMO/If Action Subsystem1/First Order Filter ==
  input : Inport
  Add : Sum  Inputs=+-
  Add3 : Sum  AccumDataTypeStr=single
  Constant : Constant  OutDataTypeStr=single  SampleTime=-1
  Data Store Read1 : DataStoreRead  DataStoreName=n_Filter
  Data Store Read2 : DataStoreRead  DataStoreName=SMO_Filter
  Gain : Gain  Gain=2*pi*Ts_20KHz*20
  Gain1 : Gain  Gain=2*pi*Ts_20KHz*20
  Product : Product
  Product1 : Product
  Unit Delay3 : UnitDelay  SampleTime=-1  HasFrameUpgradeWarning=on
  "output " : Outport
  wires:
  input/1 -> Product/1
  Product/1 -> Add3/1
  Product1/1 -> Unit Delay3/1
  Add3/1 -> Product1/1, "output "/1
  Unit Delay3/1 -> Add3/2
  Data Store Read2/1 -> Gain/1
  Gain/1 -> Product/2
  Data Store Read1/1 -> Gain1/1
  Add/1 -> Product1/2
  Gain1/1 -> Add/2
  Constant/1 -> Add/1

== system Fuel_Pump_V3_1_20201113_20KHz/Motor_Control/Main Case /AD2S1210/SMA_SMO/PLL/PLL_PI  ==
  Ref : Inport
  Data Store Read : DataStoreRead  DataStoreName=SMO_KP
  Data Store Read1 : DataStoreRead  DataStoreName=SMO_uin
  Data Store Write1 : DataStoreWrite  DataStoreName=SMO_uin
  "Integral " : Subsystem
  Product : Product  OutDataTypeStr=Inherit: Same as first input
  Sum1 : Sum
  Out : Outport
  wires:
  Data Store Read1/1 -> "Integral "/1(OLD_UI)
  Product/1 -> Sum1/1
  Data Store Read/1 -> Product/2
  Ref/1 -> "Integral "/2(UP), Product/1
  "Integral "/1(UI) -> Data Store Write1/1, Sum1/2
  Sum1/1 -> Out/1

== system Fuel_Pump_V3_1_20201113_20KHz/Motor_Control/Main Case /Position Loop Mode/If Action Subsystem/PID_Loop/UI_REG3 ==
  OLD_UI_REG3 : Inport
  up_reg3 : Inport  Port=2
  Data Store Read : DataStoreRead  DataStoreName=PK_Kin
  Data Type Conversion : DataTypeConversion
  Product : Product  OutDataTypeStr=Inherit: Same as first input
  Sum1 : Sum  OutDataTypeStr=fixdt(1,32,16)
  UI_REG1 : Outport
  wires:
  Data Type Conversion/1 -> Product/1
  Data Store Read/1 -> Data Type Conversion/1
  up_reg3/1 -> Product/2
  Sum1/1 -> UI_REG1/1
  Product/1 -> Sum1/2
  OLD_UI_REG3/1 -> Sum1/1

== system Fuel_Pump_V3_1_20201113_20KHz/Motor_Control/Main Case /Position Loop Mode/If Action Subsystem/PID_Speed/UI_REG3 ==
  OLD_UI_REG3 : Inport
  up_reg3 : Inport  Port=2
  Data Store Read : DataStoreRead  DataStoreName=PK_Kin
  Data Type Conversion : DataTypeConversion
  Product : Product  OutDataTypeStr=Inherit: Same as first input
  Sum1 : Sum  OutDataTypeStr=fixdt(1,32,16)
  UI_REG1 : Outport
  wires:
  OLD_UI_REG3/1 -> Sum1/1
  Product/1 -> Sum1/2
  Sum1/1 -> UI_REG1/1
  up_reg3/1 -> Product/2
  Data Store Read/1 -> Data Type Conversion/1
  Data Type Conversion/1 -> Product/1

== system Fuel_Pump_V3_1_20201113_20KHz/Motor_Control/Main Case /Speed Loop Mode/If Action Subsystem/PID_n /Integral  ==
  OLD_UI : Inport
  UP : Inport  Port=2
  Data Store Read2 : DataStoreRead  DataStoreName=PK_Kin
  Gain : Gain  Gain=Ts_1kHz
  Product1 : Product  OutDataTypeStr=Inherit: Same as first input
  Sum3 : Sum
  UI : Outport
  wires:
  Sum3/1 -> UI/1
  UP/1 -> Product1/2
  Product1/1 -> Sum3/2
  OLD_UI/1 -> Sum3/1
  Data Store Read2/1 -> Gain/1
  Gain/1 -> Product1/1

== system Fuel_Pump_V3_1_20201113_20KHz/Motor_Control/Main Case /AD2S1210/SMA_SMO/PLL/PLL_PI /Integral  ==
  OLD_UI : Inport
  UP : Inport  Port=2
  Data Store Read2 : DataStoreRead  DataStoreName=SMO_KI
  Gain : Gain  Gain=Ts_20KHz
  Product1 : Product  OutDataTypeStr=Inherit: Same as first input
  Sum3 : Sum
  UI : Outport
  wires:
  Sum3/1 -> UI/1
  UP/1 -> Product1/2
  Product1/1 -> Sum3/2
  OLD_UI/1 -> Sum3/1
  Data Store Read2/1 -> Gain/1
  Gain/1 -> Product1/1

== matlab function Fuel_Pump_V3_1_20201113_20KHz/Motor_Control/Main Case /Speed Loop Mode/MATLAB Function ==
  events: SPEED_PI output FUNCTION_CALL_EVENT
function  Count()
persistent count; 
if isempty(count)
    count = 0;
end

count = count + 1;
if(count >= 20)
    SPEED_PI;
    count = 0;
end

end

== matlab function Fuel_Pump_V3_1_20201113_20KHz/Motor_Control/Main Case /MATLAB Function ==
  data: U1 input; V1 input; W1 input; Protect_Flag data_store_memory; Stop data_store_memory; RMS_Count data_store_memory
function Protect(U1,V1,W1)
global Protect_Flag Stop RMS_Count;
if(abs(U1)>60||abs(V1)>60||abs(W1)>60)
    RMS_Count = RMS_Count + uint16(1);
    if(RMS_Count >= uint16(5))
        Protect_Flag = uint16(2);
    end
else
    RMS_Count = uint16(0);
end
if(abs(U1)>85||abs(V1)>85||abs(W1)>85)
    Protect_Flag = uint16(1);
end
% if(abs(U1)>0.6||abs(V1)>0.6||abs(W1)>0.6)
%     RMS_Count = RMS_Count + uint16(1);
% end
% if(RMS_Count > 20)
%     Protect_Flag = uint16(2);
% end
if(Protect_Flag ~= uint16(0))
     Stop = uint16(1);
end

end

== matlab function Fuel_Pump_V3_1_20201113_20KHz/Motor_Control/Main Case /AD2S1210/If Action Subsystem/RAW_DATA2Angle  ==
  data: Raw_Data input; Angle_out output; Mech_Theta_out output; Mid_Position input
function [Angle_out,Mech_Theta_out] = Raw_Data2Angle(Raw_Data,Mid_Position)
    Angle = single(Mid_Position) - single(Raw_Data);
    if(Angle < 0)
        Angle = Angle + 65535;
    end
    Mech_Theta = single(Angle)*(single(1.5259e-5));
    Angle = single(Angle)*single(4)*(single(1.5259e-5));
    Angle = mod(Angle,single(1));
    Mech_Theta = mod(Mech_Theta,single(1));
    Angle_out = Angle;
    Mech_Theta_out = Mech_Theta;
end

== matlab function Fuel_Pump_V3_1_20201113_20KHz/Motor_Control/Main Case /Current_PI/MATLAB Function1 ==
  data: Ud input; Uq input; Ud_out output; Us_out output; Uq_out output; ControlMode data_store_memory; Ud_VVF data_store_memory; Uq_VVF data_store_memory; MotorPara_Base_V parameter
function [Ud_out,Us_out,Uq_out] = Over_Modulation(Ud,Uq,MotorPara_Base_V)
global ControlMode Uq_VVF Ud_VVF;
Us = sqrt(Ud*Ud+Uq*Uq);
Us_out = Us;
if(Us>MotorPara_Base_V)
    Ud_out_temp = Ud/Us;
    Uq_out_temp = Uq/Us;
else
    Ud_out_temp = Ud;
    Uq_out_temp = Uq;
end
    
if(ControlMode == 4)
    Ud_out = Ud_VVF;
    Uq_out = Uq_VVF;
else
    Ud_out = Ud_out_temp;
    Uq_out = Uq_out_temp;
end
    
end

== matlab function Fuel_Pump_V3_1_20201113_20KHz/Motor_Control/Main Case /SVPWM/MATLAB Function ==
  data: alpha input; ta output; beta input; tb output; tc output
function [ta,tb,tc] = SVPWM(alpha,beta)

temp1=beta;
temp2=0.5*beta+0.86603*alpha;
temp3=temp2-temp1;

VecSector=3;
if(temp2>0)
    VecSector=VecSector-1;
end
if(temp3>0)
    VecSector=VecSector-1;
end
if(temp1<0)
    VecSector=7-VecSector;
end

switch VecSector
    case 1
        ta=temp2;
        tb=temp1-temp3;
        tc=-temp2;
    case 2
        ta=temp3+temp2;
        tb=temp1;
        tc=-temp1;
    case 3
        ta=temp3;
        tb=-temp3;
        tc=-(temp1+temp2);
    case 4
        ta=temp2;
        tb=temp1-temp3;
        tc=-temp2;
    case 5
        ta=temp3+temp2;
        tb=temp1;
        tc=-temp1;
    case 6
        ta=temp3;
        tb=-temp3;
        tc=-(temp1+temp2);
    otherwise
        ta=single(0.5);
        tb=single(0.5);
        tc=single(0.5);
end

== matlab function Fuel_Pump_V3_1_20201113_20KHz/Motor_Control/Main Case /AD2S1210/SMA_SMO/EMF Alpha/MATLAB Function ==
  data: Input input; Output output; A input; Slide input
function Output = Sigmoid(Input,A,Slide)
    Output = (2.0./(1+exp(-A*Input))-1)*Slide;
end

== matlab function Fuel_Pump_V3_1_20201113_20KHz/Motor_Control/Main Case /AD2S1210/SMA_SMO/EMF Beta/MATLAB Function ==
  data: Input input; Output output; A input; Slide input
function Output = Sigmoid(Input,A,Slide)
    Output = (2.0./(1+exp(-A*Input))-1)*Slide;
end

== matlab function Fuel_Pump_V3_1_20201113_20KHz/Motor_Control/Main Case /MATLAB Function3 ==
  data: Stop input; uin data_store_memory
function PI_Clear(Stop)
global uin
    if(Stop == uint16(1))
        uin = single(0);
    end
end

== matlab function Fuel_Pump_V3_1_20201113_20KHz/Set_nDem/MATLAB Function2 ==
  data: Target input; Set_Point output; Step input; SetpointValue data_store_memory
function Set_Point = RAMP_Control(Target,Step)
global SetpointValue;
if(Target >= SetpointValue)
    SetpointValue = SetpointValue + Step;
else
    SetpointValue = SetpointValue - Step;
end

if(SetpointValue >= single(1))
    SetpointValue = Target;
elseif(SetpointValue <= 0)
    SetpointValue = single(0);
end
Set_Point = SetpointValue;
end

== matlab function Fuel_Pump_V3_1_20201113_20KHz/Motor_Control/Main Case /Speed Loop Mode/MATLAB Function1 ==
  data: Theta_1210 input; SMO_Flag input; Theta output; Theta_SMO input
function Theta = SMO_Switch(Theta_1210,SMO_Flag,Theta_SMO)
persistent SMO_Count;
if isempty(SMO_Count)
   SMO_Count=single(0);
end
if(SMO_Flag == uint16(0))
    SMO_Count = single(0);
    Theta = Theta_1210;
else
    SMO_Count = SMO_Count + single(1);
    if(SMO_Count >= single(2000))
        SMO_Count = single(2000);
    end
     Theta = Theta_SMO*(SMO_Count/single(2000)) + Theta_1210*( (single(2000)-SMO_Count) /single(2000));
%     Theta = Theta_SMO;
end

== matlab function Fuel_Pump_V3_1_20201113_20KHz/Motor_Control/Main Case /AD2S1210/SMA_SMO/Estimated EMF_Alpha/MATLAB Function ==
  data: input input; output output; slide input; E0 input
function output = sigmoid(input,slide,E0)
output = (2.0./(1+exp(-E0*input))-1)*slide;
end

== matlab function Fuel_Pump_V3_1_20201113_20KHz/Function-Call Subsystem1/READ Temp ==
  data: AD input; TEMP output
function TEMP = READ_TEMP(AD)
    temp_AD = single(AD);
    TEMP = 1/((log(temp_AD)-log(4096-temp_AD))*0.00025316+0.00335402)-273.15;
end

== matlab function Fuel_Pump_V3_1_20201113_20KHz/Function-Call Subsystem1/READ Temp1 ==
  data: AD input; TEMP output
function TEMP = READ_TEMP(AD)
    temp_AD = single(AD);
    TEMP = 1/((log(temp_AD)-log(4096-temp_AD))*0.00025316+0.00335402)-273.15;
end

== matlab function Fuel_Pump_V3_1_20201113_20KHz/Motor_Control/Main Case /Position Loop Mode/MATLAB Function ==
  events: SPEED_PI output FUNCTION_CALL_EVENT
function  Count()
persistent count; 
if isempty(count)
    count = 0;
end

count = count + 1;
if(count >= 20)
    SPEED_PI;
    count = 0;
end

end

== matlab function Fuel_Pump_V3_1_20201113_20KHz/Motor_Control/Main Case /AD2S1210/SMA_SMO/If Action Subsystem1/MATLAB Function1 ==
  data: theta input; speed output single; theta_old input; Ts_20KHz parameter
function speed = Est_Speed(theta,theta_old, Ts_20KHz)

error = (theta - theta_old)*2*pi;
if(error > pi)
    error = error - 2*pi;
elseif(error <- pi)
	error = error + 2*pi;
end
speed = error/(Ts_20KHz*20)*30/pi/4;
% if(error>2*pi||error<-2*pi)
%     error = 0.0;
% end

end

== matlab function Fuel_Pump_V3_1_20201113_20KHz/Motor_Control/Main Case /AD2S1210/SMA_SMO/MATLAB Function ==
  data: Flag output
function Flag = Speed_Count
persistent SMO_n_Count;
if isempty(SMO_n_Count)
   SMO_n_Count=single(0);
end
if(SMO_n_Count > uint16(20))
    Flag = uint16(1);
    SMO_n_Count = single(0);
else
    Flag = uint16(0);
	SMO_n_Count = SMO_n_Count + single(1);  
end
end

== matlab function Fuel_Pump_V3_1_20201113_20KHz/SCI_TX/SCI_TX/MATLAB Function20 ==
  data: RAW_DATA input; TX_DATA output
function TX_DATA = SCI_Encoding_Res(RAW_DATA)
LSB = single(2*pi/32767);
Real_DATA = single(single(RAW_DATA)/single(65535)*single(2*pi))/LSB;
if(Real_DATA >= 0&&Real_DATA<=32767)
    SCI_Buffer = uint16(Real_DATA/single(1));
elseif(Real_DATA>32767)
    SCI_Buffer = uint16(32767);
else
    SCI_Buffer = uint16(0);
end
    TX_DATA = SCI_Buffer;
end

== matlab function Fuel_Pump_V3_1_20201113_20KHz/Motor_Control/Main Case /AD2S1210/SMA_SMO/Estimated EMF_Beta/MATLAB Function ==
  data: input input; output output; slide input; E0 input
function output = sigmoid(input,slide,E0)
output = (2.0./(1+exp(-E0*input))-1)*slide;
end

== matlab function Fuel_Pump_V3_1_20201113_20KHz/Set_nDem/MATLAB Function1 ==
  data: Target input; Set_Point output; Step input; SetpointValue data_store_memory
function Set_Point = RAMP_Control(Target,Step)
global SetpointValue;
if(abs(Target) <= single(0.25))
    if(Target >= SetpointValue)
        SetpointValue = SetpointValue + Step;
    else
        SetpointValue = SetpointValue - Step;
    end
else
    if(Target >= SetpointValue)
        SetpointValue = SetpointValue + Step/2;
    else
        SetpointValue = SetpointValue - Step/2;
    end    
end
if(abs(Target - SetpointValue) <= Step*2)
    SetpointValue = Target;
end

% if(Target>0&&SetpointValue>Target)
%     SetpointValue = Target;
% elseif(Target<=0&&SetpointValue<Target)
%     SetpointValue = Target;
% end
if(SetpointValue >= single(0))
    SetpointValue = single(0);
elseif(SetpointValue <= single(-1))
    SetpointValue = single(-1);
end
Set_Point = SetpointValue;
end

== matlab function Fuel_Pump_V3_1_20201113_20KHz/IIC_Interrupt /MATLAB Function ==
  data: TEMP_Flag data_store_memory
  events: TEMP1 output FUNCTION_CALL_EVENT; TEMP2 output FUNCTION_CALL_EVENT
function TEMP_Read
global TEMP_Flag;
    switch TEMP_Flag
        case 1
            TEMP1;
        case 2
            TEMP2;
    end
end

== matlab function Fuel_Pump_V3_1_20201113_20KHz/IIC_Interrupt /Subsystem/Temp_conv ==
  data: u1 input; y output; u2 input
function y = fcn(u1, u2)
y=single(uint16(u1)*uint16(256)+uint16(u2))*single(0.01284)-single(260);

== matlab function Fuel_Pump_V3_1_20201113_20KHz/IIC_Interrupt /Subsystem1/Temp_conv ==
  data: u1 input; y output; u2 input
function y = fcn(u1, u2)
y=single(uint16(u1)*uint16(256)+uint16(u2))*single(0.01284)-single(260);

== matlab function Fuel_Pump_V3_1_20201113_20KHz/Motor_Control/Main Case /AD2S1210/SMA_SMO/MATLAB Function1 ==
  data: Est_Alpha input; Theta output; Est_Beta input
function Theta = atan(Est_Alpha,Est_Beta)

Theta = atan2(-Est_Alpha,Est_Beta);

end

== matlab function Fuel_Pump_V3_1_20201113_20KHz/IIC_PT1000/MATLAB Function ==
  data: TEMP_Flag data_store_memory
  events: TEMP1 output FUNCTION_CALL_EVENT; TEMP2 output FUNCTION_CALL_EVENT
function temp_count
global TEMP_Flag;
persistent count;   
if isempty(count)
    count = 1;
end
count = count+1;
if(count >= 3)
	count = 1;
end

switch count
    case 1
        TEMP_Flag = uint16(1);
        TEMP1;
    case 2
        TEMP_Flag = uint16(2);
        TEMP2;
end

== matlab function Fuel_Pump_V3_1_20201113_20KHz/Motor_Control/Main Case /AD2S1210/SMA_SMO/If Action Subsystem1/Kalman_Filter ==
  data: Input input; optimal_value_out output; n_Q input; n_R input
function optimal_value_out = Kalman(Input,n_Q,n_R)
persistent Optimal_Value Deviation_Value
if isempty(Optimal_Value)
    Optimal_Value = single(0);
end
if isempty(Deviation_Value)
    Deviation_Value = single(0);
end

n_Q=1.00;																	%系统过程噪声协方差
n_R=10;																		%测量结果噪声协方差  越大每一次进行是变化越大
% System_forecast=0;                                                        %系统当前预测值定义
% deviation_forecast=0;                                                     %系统当前误差值定义
% Kalman_Gain=0;															%卡尔曼增益定义
%最优值计算
System_forecast=Optimal_Value;												%公式一
deviation_forecast=Deviation_Value+n_Q; 											%公式二
Kalman_Gain=(deviation_forecast)/(deviation_forecast+n_R);					%公式四
Optimal_Value=System_forecast+Kalman_Gain*(Input-System_forecast);			%公式三
Deviation_Value=(1-Kalman_Gain)*deviation_forecast;								%公式五
optimal_value_out=Optimal_Value	;											%返回当次预测最优值

== matlab function Fuel_Pump_V3_1_20201113_20KHz/Motor_Control/Main Case /Data Buffer /MATLAB Function1 ==
  data: ThetaSMO input; ThetaAD2S input; IqDem input; Iq input; IdDem input; Id input; Data_Buffer_ThetaSMO data_store_memory; Data_Buffer_ThetaAD2S data_store_memory; Data_Buffer_IdDem data_store_memory; Data_Buffer_IqDem data_store_memory; Data_Buffer_Id data_store_memory; Data_Buffer_Iq data_store_memory; Buffer_Flag data_store_memory
function Buff_Store(ThetaSMO,ThetaAD2S,IqDem,Iq,IdDem,Id)
    global Data_Buffer_ThetaSMO Data_Buffer_ThetaAD2S;
    global Data_Buffer_IqDem    Data_Buffer_IdDem;
    global Data_Buffer_Iq       Data_Buffer_Id;
    global Buffer_Flag;

    persistent count
    if isempty(count)
        count = single(1);
    end
    
    if(Buffer_Flag == 1)
        count = single(1);
    else
        if(count <= single(1000))
            Data_Buffer_ThetaSMO(count)     = single(ThetaSMO);
            Data_Buffer_ThetaAD2S(count)    = single(ThetaAD2S);
            Data_Buffer_IqDem(count)        = single(IqDem);
            Data_Buffer_IdDem(count)        = single(IdDem);
            Data_Buffer_Iq(count)           = single(Iq);
            Data_Buffer_Id(count)           = single(Id);
            count = count + single(1);
        else
            count = single(1);
            Buffer_Flag = uint16(1);
        end
    end
end

== matlab function Fuel_Pump_V3_1_20201113_20KHz/SCI_TX/MATLAB Function49 ==
  data: Data_SCI input; SCI_Error data_store_memory; Stop data_store_memory; MCU_IN data_store_memory; WFm data_store_memory; Protect_Flag data_store_memory; n data_store_memory; SCI_Break_Error data_store_memory
function Check(Data_SCI)
global SCI_Error Stop MCU_IN WFm Protect_Flag n;
global SCI_Break_Error;
Sum = bitand(uint16(Data_SCI(2))+uint16(Data_SCI(3))+uint16(Data_SCI(4))+uint16(Data_SCI(5))+uint16(Data_SCI(6))+uint16(Data_SCI(7))+uint16(Data_SCI(8))+uint16(Data_SCI(9)),255);
if(Sum == Data_SCI(10)&&Data_SCI(1)==8&&Data_SCI(2)==33)
	SCI_Error = uint16(0);
	Stop_temp = bitand(Data_SCI(5),2);
	if(Stop_temp == 0)
        WFm = single(0);
        if(abs(n)<=single(50))
            Stop = uint16(1);
        end
    else
        Stop = uint16(0);
        WFm = (single(Data_SCI(4))*single(255)+single(Data_SCI(3)))*single(500/32767);
	end
        MCU_IN = uint16(bitand(Data_SCI(5),1));
else
	SCI_Error = uint16(1);
end  
if(Protect_Flag ~= uint16(0))
	Stop = uint16(1);
end

if(Data_SCI(1)==255&&Data_SCI(2)==0&&Data_SCI(3)==0&&Data_SCI(4)==0&&Data_SCI(5)==0&&Data_SCI(6)==0&&Data_SCI(7)==0&&Data_SCI(8)==0&&Data_SCI(9)==0&&Data_SCI(10)==255)
    SCI_Break_Error = uint16(1);
else
    SCI_Break_Error = uint16(0);    
end
